simulink model "HDVPSG_DelayComp_NewRef_RealDrop_case1"  (R2019b)
settings: Solver=FixedStepDiscrete  StartTime=0.0  StopTime=28  FixedStep=UT.Ts_Veh  RelTol=1e-3
PostLoadFcn:
  | if any(exist('dsrtsu_mdlpostloadfcn', 'file') ~= 0), dsrtsu_mdlpostloadfcn('Execute', bdroot); end
InitFcn:
  | , if any(exist('dsmpb_private', 'file') ~= 0), dsmpb_private('dsmpb_mdlclblib', 'Init', bdroot); end,
values from neighbouring files (symbols this model uses):
  BETA_HDV_Leader = 50    [HDVPSG_DelayComp_NewRef_RealDrop_script_case1.m]
  BETA_PSG_Follower = 150    [HDVPSG_DelayComp_NewRef_RealDrop_script_case1.m]
  CtrlZone_Length = 250    [HDVPSG_DelayComp_NewRef_RealDrop_script_case1.m]
  DELTA_D_MIN = 5    [HDVPSG_DelayComp_NewRef_RealDrop_script_case1.m]
  DELTA_DR_MG_TCC = 15    [HDVPSG_DelayComp_NewRef_RealDrop_script_case1.m]
  HDV_AMAX = 1.3    [HDVPSG_DelayComp_NewRef_RealDrop_script_case1.m]
  HDV_AMIN = -2.5    [HDVPSG_DelayComp_NewRef_RealDrop_script_case1.m]
  HDV_first_v0 = 13    [HDVPSG_DelayComp_NewRef_RealDrop_script_case1.m]
  HDV_HighMu_D = 9    [HDVPSG_DelayComp_NewRef_RealDrop_script_case1.m]
  HDV_HighMu_I = 27    [HDVPSG_DelayComp_NewRef_RealDrop_script_case1.m]
  HDV_HighMu_P = 27    [HDVPSG_DelayComp_NewRef_RealDrop_script_case1.m]
  HDV_HighMu_TRFC = 0.7    [HDVPSG_DelayComp_NewRef_RealDrop_script_case1.m]
  HDV_last_v0 = 13    [HDVPSG_DelayComp_NewRef_RealDrop_script_case1.m]
  HDV_LowMu_D = 6    [HDVPSG_DelayComp_NewRef_RealDrop_script_case1.m]
  HDV_LowMu_I = 8    [HDVPSG_DelayComp_NewRef_RealDrop_script_case1.m]
  HDV_LowMu_P = 12    [HDVPSG_DelayComp_NewRef_RealDrop_script_case1.m]
  HDV_LowMu_TRFC = 0.6    [HDVPSG_DelayComp_NewRef_RealDrop_script_case1.m]
  Np_MPC = 20    [HDVPSG_DelayComp_NewRef_RealDrop_script_case1.m]
  PSG_AMAX = 3.2    [HDVPSG_DelayComp_NewRef_RealDrop_script_case1.m]
  PSG_AMIN = -6    [HDVPSG_DelayComp_NewRef_RealDrop_script_case1.m]
  PSG_end_v0 = 13    [HDVPSG_DelayComp_NewRef_RealDrop_script_case1.m]
  PSG_first_v0 = 13    [HDVPSG_DelayComp_NewRef_RealDrop_script_case1.m]
  PSG_HighMu_D = 15    [HDVPSG_DelayComp_NewRef_RealDrop_script_case1.m]
  PSG_HighMu_I = 125    [HDVPSG_DelayComp_NewRef_RealDrop_script_case1.m]
  PSG_HighMu_P = 75    [HDVPSG_DelayComp_NewRef_RealDrop_script_case1.m]
  PSG_HighMu_TRFC = 0.8    [HDVPSG_DelayComp_NewRef_RealDrop_script_case1.m]
  PSG_LowMu_D = 12    [HDVPSG_DelayComp_NewRef_RealDrop_script_case1.m]
  PSG_LowMu_I = 64    [HDVPSG_DelayComp_NewRef_RealDrop_script_case1.m]
  PSG_LowMu_P = 48    [HDVPSG_DelayComp_NewRef_RealDrop_script_case1.m]
  PSG_LowMu_TRFC = 0.7    [HDVPSG_DelayComp_NewRef_RealDrop_script_case1.m]
  PSG_middle_v0 = 13    [HDVPSG_DelayComp_NewRef_RealDrop_script_case1.m]
  Q_Leader = 1    [HDVPSG_DelayComp_NewRef_RealDrop_script_case1.m]
  Qd_dot_PSG_Follower = 2    [HDVPSG_DelayComp_NewRef_RealDrop_script_case1.m]
  Qd_PSG_Follower = 10    [HDVPSG_DelayComp_NewRef_RealDrop_script_case1.m]
  R_Leader = 20    [HDVPSG_DelayComp_NewRef_RealDrop_script_case1.m]
  R_PSG_Follower = 1    [HDVPSG_DelayComp_NewRef_RealDrop_script_case1.m]
  Recved_40_1 = Recved_Flag_Combined(47740,:)    [HDVPSG_DelayComp_NewRef_RealDrop_script_case1.m]
  Recved_40_2 = Recved_Flag_Combined(47780,:)    [HDVPSG_DelayComp_NewRef_RealDrop_script_case1.m]
  Recved_40_3 = Recved_Flag_Combined(49536,:)    [HDVPSG_DelayComp_NewRef_RealDrop_script_case1.m]
  Recved_40_4 = Recved_Flag_Combined(118106,:)    [HDVPSG_DelayComp_NewRef_RealDrop_script_case1.m]
  Rho_deltad_PSG_Follower = 1e3    (= 1000)    [HDVPSG_DelayComp_NewRef_RealDrop_script_case1.m]
  Rho_v_PSG_Follower = 1e3    (= 1000)    [HDVPSG_DelayComp_NewRef_RealDrop_script_case1.m]
  T_ADE = 0.01    [HDVPSG_DelayComp_NewRef_RealDrop_script_case1.m]
  V_MAX = 40    [HDVPSG_DelayComp_NewRef_RealDrop_script_case1.m]
  V_MIN = 0    [HDVPSG_DelayComp_NewRef_RealDrop_script_case1.m]
  VR_MG_TCC = 15    [HDVPSG_DelayComp_NewRef_RealDrop_script_case1.m]
undefined symbols (not defined in the file or in its folder): DiscIntNeverNeededParam, UT
libraries: simulink x46
(part 5 of 16)

== system HDVPSG_DelayComp_NewRef_RealDrop_case1/Subsystem1/PSG_first/Global Coordinates ==
  Heading Angle : Inport
  Vx : Inport  Port=2
  Vy : Inport  Port=3
  Add : Sum
  Discrete-Time Integrator : DiscreteIntegrator  SampleTime=UT.Ts_Veh  ICPrevOutput=DiscIntNeverNeededParam  ICPrevScaledInput=DiscIntNeverNeededParam
  Discrete-Time Integrator1 : DiscreteIntegrator  SampleTime=UT.Ts_Veh  ICPrevOutput=DiscIntNeverNeededParam  ICPrevScaledInput=DiscIntNeverNeededParam
  Math Function : Math  Operator=square  SaturateOnIntegerOverflow=on
  Math Function1 : Math  Operator=square  SaturateOnIntegerOverflow=on
  Product{,1..3} (4 alike) : Product
  Sign : Signum
  Sign1 : Signum
  Sqrt : Sqrt  Operator=signedSqrt  SaturateOnIntegerOverflow=on
  Trigonometric Function : Trigonometry
  Trigonometric Function1 : Trigonometry  Operator=cos
  X : Outport  VectorParamsAs1DForOutWhenUnconnected=off
  Y : Outport  Port=2  VectorParamsAs1DForOutWhenUnconnected=off
  wires:
  Product3/1 -> Add/2
  Sign1/1 -> Product3/2
  Math Function1/1 -> Product3/1
  Product2/1 -> Add/1
  Sign/1 -> Product2/2
  Math Function/1 -> Product2/1
  Discrete-Time Integrator/1 -> Y/1
  Discrete-Time Integrator1/1 -> X/1
  Product1/1 -> Discrete-Time Integrator/1
  Product/1 -> Discrete-Time Integrator1/1
  Trigonometric Function/1 -> Product1/1
  Trigonometric Function1/1 -> Product/1
  Sqrt/1 -> Product/2, Product1/2
  Heading Angle/1 -> Trigonometric Function/1, Trigonometric Function1/1
  Add/1 -> Sqrt/1
  Vy/1 -> Sign1/1, Math Function1/1
  Vx/1 -> Sign/1, Math Function/1

== system HDVPSG_DelayComp_NewRef_RealDrop_case1/Subsystem1/PSG_first/left//right wheel steer ==
  steering wheel angle deg : Inport
  Deadband Deg : DeadZone  LowerValue=-2  UpperValue=2  SaturateOnIntegerOverflow=on
  Gain : Gain  Gain=0.9
  Gain1 : Gain  Gain=0.9
  Left wheel rack displacement to ground steering angle1 : Lookup_n-D  NumberOfTableDimensions=1  BreakpointsForDimension1=|  Table=|  RndMeth=Simplest  InputSameDT=on
      | [-83.31
      | -80.10576923
      | -77.13888889
      | -74.38392857
      | -71.81896552
      | -69.425
      | -67.18548387
      | -65.0859375
      | -63.11363636
      | -61.25735294
      | -59.50714286
      | -57.85416667
      | -56.29054054
      | -54.80921053
      | -53.40384615
      | -52.06875
      | -50.79878049
      | -49.58928571
      | -48.43604651
      | -47.33522727
      | -46.28333333
      | -45.27717391
      | -44.31382979
      | -43.390625
      | -42.50510204
      | -41.655
      | 0
      | 41.655
      | 42.50510204
      | 43.390625
      | 44.31382979
      | 45.27717391
      | 46.28333333
      | 47.33522727
      | 48.43604651
      | 49.58928571
      | 50.79878049
      | 52.06875
      | 53.40384615
      | 54.80921053
      | 56.29054054
      | 57.85416667
      | 59.50714286
      | 61.25735294
      | 63.11363636
      | 65.0859375
      | 67.18548387
      | 69.425
      | 71.81896552
      | 74.38392857
      | 77.13888889
      | 80.10576923
      | 83.31
      | ]
      | [-39.37720355
      | -37.63494871
      | -36.07707064
      | -34.67025898
      | -33.38971041
      | -32.21639355
      | -31.13534711
      | -30.13457154
      | -29.20427963
      | -28.33637359
      | -27.52407048
      | -26.76162747
      | -26.04413644
      | -25.36736764
      | -24.72764882
      | -24.12177053
      | -23.54691095
      | -23.00057556
      | -22.48054833
      | -21.98485165
      | -21.51171342
      | -21.05953958
      | -20.62689117
      | -20.21246499
      | -19.81507719
      | -19.43364926
      | 0
      | 23.71741561
      | 24.27669186
      | 24.86323253
      | 25.47909206
      | 26.1265372
      | 26.80807528
      | 27.52648702
      | 28.28486498
      | 29.08665866
      | 29.93572777
      | 30.83640531
      | 31.7935729
      | 32.81275112
      | 33.9002085
      | 35.06309421
      | 36.30960068
      | 37.64916478
      | 39.09271935
      | 40.65301137
      | 42.34501024
      | 44.1864403
      | 46.19848973
      | 48.40677775
      | 50.84271532
      | 53.54549481
      | 56.56514507
      | ]
  Right wheel rack displacement to ground steering angle : Lookup_n-D  NumberOfTableDimensions=1  BreakpointsForDimension1=|  Table=|  RndMeth=Simplest  InputSameDT=on
      | [-83.31
      | -80.10576923
      | -77.13888889
      | -74.38392857
      | -71.81896552
      | -69.425
      | -67.18548387
      | -65.0859375
      | -63.11363636
      | -61.25735294
      | -59.50714286
      | -57.85416667
      | -56.29054054
      | -54.80921053
      | -53.40384615
      | -52.06875
      | -50.79878049
      | -49.58928571
      | -48.43604651
      | -47.33522727
      | -46.28333333
      | -45.27717391
      | -44.31382979
      | -43.390625
      | -42.50510204
      | -41.655
      | 0
      | 41.655
      | 42.50510204
      | 43.390625
      | 44.31382979
      | 45.27717391
      | 46.28333333
      | 47.33522727
      | 48.43604651
      | 49.58928571
      | 50.79878049
      | 52.06875
      | 53.40384615
      | 54.80921053
      | 56.29054054
      | 57.85416667
      | 59.50714286
      | 61.25735294
      | 63.11363636
      | 65.0859375
      | 67.18548387
      | 69.425
      | 71.81896552
      | 74.38392857
      | 77.13888889
      | 80.10576923
      | 83.31
      | ]
      | [-56.56514507
      | -53.54549481
      | -50.84271532
      | -48.40677775
      | -46.19848973
      | -44.1864403
      | -42.34501024
      | -40.65301137
      | -39.09271935
      | -37.64916478
      | -36.30960068
      | -35.06309421
      | -33.9002085
      | -32.81275112
      | -31.7935729
      | -30.83640531
      | -29.93572777
      | -29.08665866
      | -28.28486498
      | -27.52648702
      | -26.80807528
      | -26.1265372
      | -25.47909206
      | -24.86323253
      | -24.27669186
      | -23.71741561
      | 0
      | 19.43364926
      | 19.81507719
      | 20.21246499
      | 20.62689117
      | 21.05953958
      | 21.51171342
      | 21.98485165
      | 22.48054833
      | 23.00057556
      | 23.54691095
      | 24.12177053
      | 24.72764882
      | 25.36736764
      | 26.04413644
      | 26.76162747
      | 27.52407048
      | 28.33637359
      | 29.20427963
      | 30.13457154
      | 31.13534711
      | 32.21639355
      | 33.38971041
      | 34.67025898
      | 36.07707064
      | 37.63494871
      | 39.37720355
      | ]
  steering wheel angle (pinion) to rack dispacement : Lookup_n-D  NumberOfTableDimensions=1  BreakpointsForDimension1=|  Table=|  RndMeth=Simplest  InputSameDT=on
      BreakpointsForDimension1=|
      | [-807.1596203
      | -767.526082
      | -732.1745847
      | -700.3549602
      | -671.5005069
      | -645.1711331
      | -621.017417
      | -598.7568399
      | -578.1574816
      | -559.0264878
      | -541.2017003
      | -524.5454483
      | -508.9398532
      | -494.2832202
      | -480.4872231
      | -467.4746805
      | -455.1777777
      | -443.5366317
      | -432.4981203
      | -422.0149202
      | -412.0447096
      | -402.5495034
      | -393.495094
      | -384.8505798
      | -376.5879637
      | -368.6818104
      | 0
      | 368.6818104
      | 376.5879637
      | 384.8505798
      | 393.495094
      | 402.5495034
      | 412.0447096
      | 422.0149202
      | 432.4981203
      | 443.5366317
      | 455.1777777
      | 467.4746805
      | 480.4872231
      | 494.2832202
      | 508.9398532
      | 524.5454483
      | 541.2017003
      | 559.0264878
      | 578.1574816
      | 598.7568399
      | 621.017417
      | 645.1711331
      | 671.5005069
      | 700.3549602
      | 732.1745847
      | 767.526082
      | 807.1596203
      | ]
      Table=|
      | [-83.31
      | -80.10576923
      | -77.13888889
      | -74.38392857
      | -71.81896552
      | -69.425
      | -67.18548387
      | -65.0859375
      | -63.11363636
      | -61.25735294
      | -59.50714286
      | -57.85416667
      | -56.29054054
      | -54.80921053
      | -53.40384615
      | -52.06875
      | -50.79878049
      | -49.58928571
      | -48.43604651
      | -47.33522727
      | -46.28333333
      | -45.27717391
      | -44.31382979
      | -43.390625
      | -42.50510204
      | -41.655
      | 0
      | 41.655
      | 42.50510204
      | 43.390625
      | 44.31382979
      | 45.27717391
      | 46.28333333
      | 47.33522727
      | 48.43604651
      | 49.58928571
      | 50.79878049
      | 52.06875
      | 53.40384615
      | 54.80921053
      | 56.29054054
      | 57.85416667
      | 59.50714286
      | 61.25735294
      | 63.11363636
      | 65.0859375
      | 67.18548387
      | 69.425
      | 71.81896552
      | 74.38392857
      | 77.13888889
      | 80.10576923
      | 83.31
      | ]
  Right wheel steer ground (deg) : Outport  VectorParamsAs1DForOutWhenUnconnected=off
  Left wheel steer ground (deg) : Outport  Port=2  VectorParamsAs1DForOutWhenUnconnected=off
  wires:
  Deadband Deg/1 -> steering wheel angle (pinion) to rack dispacement/1
  Gain1/1 -> Left wheel steer ground (deg)/1
  Gain/1 -> Right wheel steer ground (deg)/1
  Left wheel rack displacement to ground steering angle1/1 -> Gain1/1
  Right wheel rack displacement to ground steering angle/1 -> Gain/1
  steering wheel angle (pinion) to rack dispacement/1 -> Right wheel rack displacement to ground steering angle/1, Left wheel rack displacement to ground steering angle1/1
  steering wheel angle deg/1 -> Deadband Deg/1

== system HDVPSG_DelayComp_NewRef_RealDrop_case1/Subsystem2/PSG_first/Body Fixed Vehicle Dynamics ==
  Tdf : Inport
  Brake : Inport  Port=2
  deltaFR : Inport  Port=3
  deltaFL : Inport  Port=4
  slope : Inport  Port=5
  TRFC : Inport  Port=6
  V_ini : Inport  Port=7
  yaw_ini : Inport  Port=8
  vy_ini : Inport  Port=9
  8dof_vehicle : Subsystem
  Brakes : Subsystem
  Bus Creator{,2..4} (4 alike) : BusCreator  Inputs=4
  Bus Creator1 : BusCreator  Inputs=8
  Bus Creator5 : BusCreator  Inputs=3
  Bus Selector : BusSelector  OutputSignals=signal1,signal2,signal3,signal4
  Constant : Constant  Value=0
  Constant1 : Constant  Value=0
  Driving Resistance Subsystem : Subsystem
  Fz : Subsystem
  Magic Formula Tire Model1 : Subsystem
  "Tire Longitudinal Center Speed " : Subsystem
  Tire Sideslip Angle : Subsystem
  Unit Delay : UnitDelay  SampleTime=UT.Ts_Veh  HasFrameUpgradeWarning=on
  Unit Delay1 : UnitDelay  SampleTime=UT.Ts_Veh  HasFrameUpgradeWarning=on
  deltaFL1 : InportShadow  Port=4
  deltaFL2 : InportShadow  Port=4
  deltaFR1 : InportShadow  Port=3
  deltaFR2 : InportShadow  Port=3
  lamda slip ratio : Subsystem
  omegafl : Outport  VectorParamsAs1DForOutWhenUnconnected=off
  omegafr : Outport  Port=2  VectorParamsAs1DForOutWhenUnconnected=off
  omegarl : Outport  Port=3  VectorParamsAs1DForOutWhenUnconnected=off
  omegarr : Outport  Port=4  VectorParamsAs1DForOutWhenUnconnected=off
  ax : Outport  Port=5  VectorParamsAs1DForOutWhenUnconnected=off
  Vx : Outport  Port=6  VectorParamsAs1DForOutWhenUnconnected=off
  "Yaw Rate " : Outport  Port=7  VectorParamsAs1DForOutWhenUnconnected=off
  Yaw Angle : Outport  Port=8  VectorParamsAs1DForOutWhenUnconnected=off
  ay : Outport  Port=9  VectorParamsAs1DForOutWhenUnconnected=off
  Vy : Outport  Port=10  VectorParamsAs1DForOutWhenUnconnected=off
  Beta : Outport  Port=11  VectorParamsAs1DForOutWhenUnconnected=off
  Sideslip Angle Alpha : Outport  Port=12  VectorParamsAs1DForOutWhenUnconnected=off
  wires:
  8dof_vehicle/15(Roll Rate) -> Fz/9(roll rate)
  vy_ini/1 -> 8dof_vehicle/14(vy_ini)
  yaw_ini/1 -> 8dof_vehicle/13(yaw_ini)
  V_ini/1 -> 8dof_vehicle/12(V_ini)
  TRFC/1 -> Magic Formula Tire Model1/2(TRFC)
  Bus Creator/1 -> Bus Selector/1
  Tdf/1 -> 8dof_vehicle/1(Tdf)
  8dof_vehicle/1(omegafl) -> omegafl/1, lamda slip ratio/1(omegafl)
  8dof_vehicle/2(omegafr) -> omegafr/1, lamda slip ratio/2(omegafr)
  8dof_vehicle/3(omegarl) -> omegarl/1, lamda slip ratio/3(omegarl)
  8dof_vehicle/4(omegarr) -> omegarr/1, lamda slip ratio/4(omegarr)
  8dof_vehicle/8(Yaw angle) -> Yaw Angle/1
  Bus Creator1/1 -> 8dof_vehicle/6(In7)
  8dof_vehicle/10(Vy) -> Vy/1, Tire Sideslip Angle/1(Vy), "Tire Longitudinal Center Speed "/2(Vy)
  Magic Formula Tire Model1/2(Fy_FL) -> Bus Creator1/2
  Magic Formula Tire Model1/1(Fx_FL) -> Bus Creator1/1
  Fz/4(Fzrr) -> Bus Creator3/4
  Fz/3(Fzrl) -> Bus Creator3/3
  Fz/2(Fzfr) -> Bus Creator3/2
  Fz/1(Fzfl) -> Bus Creator3/1
  Bus Creator2/1 -> Bus Creator5/1, Brakes/1(lambda)  "lamda"
  Bus Creator4/1 -> Bus Creator5/3  "alpha"
  Bus Creator5/1 -> Magic Formula Tire Model1/1(VehState)
  Tire Sideslip Angle/4(alpha_rr: rad) -> Bus Creator4/4
  Tire Sideslip Angle/3(alpha_rl: rad) -> Bus Creator4/3
  Tire Sideslip Angle/1(alpha_fl: rad) -> Bus Creator4/1, Sideslip Angle Alpha/1
  Tire Sideslip Angle/2(alpha_fr: rad) -> Bus Creator4/2
  "Tire Longitudinal Center Speed "/4(Vwrr) -> Bus Creator/4
  "Tire Longitudinal Center Speed "/2(Vwfr) -> Bus Creator/2
  "Tire Longitudinal Center Speed "/1(Vwfl) -> Bus Creator/1
  "Tire Longitudinal Center Speed "/3(Vwrl) -> Bus Creator/3
  Bus Selector/1 -> lamda slip ratio/5(Vwfl)  "<signal1>"
  Bus Selector/2 -> lamda slip ratio/6(Vwfr)  "<signal2>"
  Bus Selector/3 -> lamda slip ratio/7(Vwrl)  "<signal3>"
  Bus Selector/4 -> lamda slip ratio/8(Vwrr)  "<signal4>"
  Driving Resistance Subsystem/2(Fr) -> 8dof_vehicle/8(Fr)
  deltaFL/1 -> lamda slip ratio/9(deltaFL)  "deltaw"
  deltaFL1/1 -> Tire Sideslip Angle/4(deltaFL)  "deltaw"
  8dof_vehicle/9(ay) -> ay/1, Unit Delay1/1
  8dof_vehicle/11("Veh Sideslip, Beta") -> "Tire Longitudinal Center Speed "/4(VehSideSlip Beta), Beta/1, Tire Sideslip Angle/6(Beta)
  8dof_vehicle/6(Vx) -> Vx/1, Driving Resistance Subsystem/1(Vx), Tire Sideslip Angle/3(Vx), "Tire Longitudinal Center Speed "/1(Vx)
  8dof_vehicle/7(Yaw Rate) -> "Yaw Rate "/1, Tire Sideslip Angle/2(Yaw Rate), "Tire Longitudinal Center Speed "/3(YawRate)
  slope/1 -> 8dof_vehicle/9(slope)
  Constant1/1 -> Fz/6(bank angle)
  Driving Resistance Subsystem/1(Fax) -> Fz/1(Fa), 8dof_vehicle/7(Fax)
  Constant/1 -> Fz/3(slope)
  8dof_vehicle/5(ax) -> ax/1, Unit Delay/1
  deltaFL2/1 -> 8dof_vehicle/10(deltaFL)  "deltaw"
  Magic Formula Tire Model1/5(Fx_RL) -> Bus Creator1/5
  Magic Formula Tire Model1/7(Fx_RR) -> Bus Creator1/7
  Magic Formula Tire Model1/8(Fy_RR) -> Bus Creator1/8
  Magic Formula Tire Model1/6(Fy_RL) -> Bus Creator1/6
  Magic Formula Tire Model1/3(Fx_FR) -> Bus Creator1/3
  Magic Formula Tire Model1/4(Fy_FR) -> Bus Creator1/4
  Unit Delay1/1 -> Fz/5(ay)
  Unit Delay/1 -> Fz/2(ax)
  lamda slip ratio/1(lamdafl) -> Bus Creator2/1
  lamda slip ratio/2(lamdafr) -> Bus Creator2/2
  lamda slip ratio/3(lamdarl) -> Bus Creator2/3
  lamda slip ratio/4(lamdarr) -> Bus Creator2/4
  deltaFR/1 -> lamda slip ratio/10(deltaFR)
  deltaFR1/1 -> Tire Sideslip Angle/5(deltaFR1)
  deltaFR2/1 -> 8dof_vehicle/11(deltaRL)
  Bus Creator3/1 -> Bus Creator5/2
  8dof_vehicle/13(Pitch_rate) -> Fz/8(pitch rate)
  8dof_vehicle/12(Pitch) -> Fz/4(pitch angle)
  8dof_vehicle/14("Roll ") -> Fz/7(roll angle)
  Brake/1 -> Brakes/2(brake postion)
  Brakes/1(Tbfl) -> 8dof_vehicle/2(Tbfl)
  Brakes/2(Tbfr) -> 8dof_vehicle/3(Tbfr)
  Brakes/3(Tbrl) -> 8dof_vehicle/4(Tbrl)
  Brakes/4(Tbrr) -> 8dof_vehicle/5(Tbrr)

== system HDVPSG_DelayComp_NewRef_RealDrop_case1/Subsystem2/PSG_first/Cruise Speed Control ==
  Vx : Inport
  Vxr : Inport  Port=2
  PID_P : Inport  Port=3
  PID_I : Inport  Port=4
  PID_D : Inport  Port=5
  Constant : Constant  Value=100
  Gain : Gain  Gain=2
  PID Controller : simulink/Continuous/PID Controller  Controller=PID  Form=Parallel  TimeDomain=Discrete-time  SampleTime=UT.Ts_Veh  IntegratorMethod=Forward Euler  FilterMethod=Forward Euler  ControllerParametersSource=external  P=UT.PID_P_PSG  I=UT.PID_I_PSG  D=UT.PID_D_PSG  UseFilter=on  N=100  TunerSelectOption=Transfer Function Based (PID Tuner App)  InitialConditionSource=internal  InitialConditionForIntegrator=0  InitialConditionForFilter=0  DifferentiatorICPrevScaledInput=0  ExternalReset=none  TrackingMode=off  Kt=1  LimitOutput=off  UpperSaturationLimit=inf  LowerSaturationLimit=-inf  LinearizeAsGain=on  AntiWindupMode=none  Kb=1  POutMin=[]  POutMax=[]  IOutMin=[]  IOutMax=[]  DOutMin=[]  DOutMax=[]  NOutMin=[]  NOutMax=[]  SumOutMin=[]  SumOutMax=[]  SaturationOutMin=[]  SaturationOutMax=[]  PParamMin=[]  PParamMax=[]  IParamMin=[]  IParamMax=[]  DParamMin=[]  DParamMax=[]  NParamMin=[]  NParamMax=[]  KbParamMin=[]  KbParamMax=[]  KtParamMin=[]  KtParamMax=[]  KbOutMin=[]  KbOutMax=[]  KtOutMin=[]  KtOutMax=[]  IntegratorOutMin=[]  IntegratorOutMax=[]  FilterOutMin=[]  FilterOutMax=[]  SumI1OutMin=[]  SumI1OutMax=[]  SumI2OutMin=[]  SumI2OutMax=[]  SumI3OutMin=[]  SumI3OutMax=[]  SumI4OutMin=[]  SumI4OutMax=[]  SumDOutMin=[]  SumDOutMax=[]  DifferentiatorOutMin=[]  DifferentiatorOutMax=[]  FilterDiffOutCoefMin=[]  FilterDiffOutCoefMax=[]  ReciprocalOutMin=[]  ReciprocalOutMax=[]  SumDenOutMin=[]  SumDenOutMax=[]  SumNumOutMin=[]  SumNumOutMax=[]  DivideOutMin=[]  DivideOutMax=[]  IntegratorContinuousStateAttributes=''  IntegratorStateMustResolveToSignalObject=off  IntegratorRTWStateStorageClass=Auto  FilterContinuousStateAttributes=''  FilterStateMustResolveToSignalObject=off  FilterRTWStateStorageClass=Auto  ParallelPVariant=ExternalParameters  IdealPVariant=Disabled  IVariant=ExternalParameters  DVariant=ExternalParameters  IntegratorVariant=Discrete  SatVariant=Disabled  AWVariant=Passthrough  PCopyVariant=Disabled  TRVariant=Disabled  FdbkBlocksVariant=Forward  IdealPFdbkVariant=Disabled  SatFdbkVariant=Disabled  DerivativeFilterVariant=ForwardEulerFilter  NVariant=ExternalParameters  NCopyVariant=Disabled  FilterICVariant=InternalICsFilter  IntegratorICVariant=InternalICs  ExternalResetVariant=Disabled  TRSumVariant=Passthrough  SumFdbkVariant=Disabled  SumVariant=Sum_PID
  Subtract : Sum  Inputs=-+
  Throttle : Outport  VectorParamsAs1DForOutWhenUnconnected=off
  wires:
  PID_D/1 -> PID Controller/4
  PID_I/1 -> PID Controller/3
  PID_P/1 -> PID Controller/2
  Constant/1 -> PID Controller/5
  PID Controller/1 -> Gain/1
  Subtract/1 -> PID Controller/1
  Gain/1 -> Throttle/1
  Vxr/1 -> Subtract/2
  Vx/1 -> Subtract/1

== system HDVPSG_DelayComp_NewRef_RealDrop_case1/Subsystem2/PSG_first/Global Coordinates ==
  Heading Angle : Inport
  Vx : Inport  Port=2
  Vy : Inport  Port=3
  Add : Sum
  Discrete-Time Integrator : DiscreteIntegrator  SampleTime=UT.Ts_Veh  ICPrevOutput=DiscIntNeverNeededParam  ICPrevScaledInput=DiscIntNeverNeededParam
  Discrete-Time Integrator1 : DiscreteIntegrator  SampleTime=UT.Ts_Veh  ICPrevOutput=DiscIntNeverNeededParam  ICPrevScaledInput=DiscIntNeverNeededParam
  Math Function : Math  Operator=square  SaturateOnIntegerOverflow=on
  Math Function1 : Math  Operator=square  SaturateOnIntegerOverflow=on
  Product{,1..3} (4 alike) : Product
  Sign : Signum
  Sign1 : Signum
  Sqrt : Sqrt  Operator=signedSqrt  SaturateOnIntegerOverflow=on
  Trigonometric Function : Trigonometry
  Trigonometric Function1 : Trigonometry  Operator=cos
  X : Outport  VectorParamsAs1DForOutWhenUnconnected=off
  Y : Outport  Port=2  VectorParamsAs1DForOutWhenUnconnected=off
  wires:
  Vx/1 -> Math Function/1, Sign/1
  Vy/1 -> Math Function1/1, Sign1/1
  Add/1 -> Sqrt/1
  Heading Angle/1 -> Trigonometric Function1/1, Trigonometric Function/1
  Sqrt/1 -> Product1/2, Product/2
  Trigonometric Function1/1 -> Product/1
  Trigonometric Function/1 -> Product1/1
  Product/1 -> Discrete-Time Integrator1/1
  Product1/1 -> Discrete-Time Integrator/1
  Discrete-Time Integrator1/1 -> X/1
  Discrete-Time Integrator/1 -> Y/1
  Math Function/1 -> Product2/1
  Sign/1 -> Product2/2
  Product2/1 -> Add/1
  Math Function1/1 -> Product3/1
  Sign1/1 -> Product3/2
  Product3/1 -> Add/2

== system HDVPSG_DelayComp_NewRef_RealDrop_case1/Subsystem2/PSG_first/left//right wheel steer ==
  steering wheel angle deg : Inport
  Deadband Deg : DeadZone  LowerValue=-2  UpperValue=2  SaturateOnIntegerOverflow=on
  Gain : Gain  Gain=0.9
  Gain1 : Gain  Gain=0.9
  Left wheel rack displacement to ground steering angle1 : Lookup_n-D  NumberOfTableDimensions=1  BreakpointsForDimension1=|  Table=|  RndMeth=Simplest  InputSameDT=on
      | [-83.31
      | -80.10576923
      | -77.13888889
      | -74.38392857
      | -71.81896552
      | -69.425
      | -67.18548387
      | -65.0859375
      | -63.11363636
      | -61.25735294
      | -59.50714286
      | -57.85416667
      | -56.29054054
      | -54.80921053
      | -53.40384615
      | -52.06875
      | -50.79878049
      | -49.58928571
      | -48.43604651
      | -47.33522727
      | -46.28333333
      | -45.27717391
      | -44.31382979
      | -43.390625
      | -42.50510204
      | -41.655
      | 0
      | 41.655
      | 42.50510204
      | 43.390625
      | 44.31382979
      | 45.27717391
      | 46.28333333
      | 47.33522727
      | 48.43604651
      | 49.58928571
      | 50.79878049
      | 52.06875
      | 53.40384615
      | 54.80921053
      | 56.29054054
      | 57.85416667
      | 59.50714286
      | 61.25735294
      | 63.11363636
      | 65.0859375
      | 67.18548387
      | 69.425
      | 71.81896552
      | 74.38392857
      | 77.13888889
      | 80.10576923
      | 83.31
      | ]
      | [-39.37720355
      | -37.63494871
      | -36.07707064
      | -34.67025898
      | -33.38971041
      | -32.21639355
      | -31.13534711
      | -30.13457154
      | -29.20427963
      | -28.33637359
      | -27.52407048
      | -26.76162747
      | -26.04413644
      | -25.36736764
      | -24.72764882
      | -24.12177053
      | -23.54691095
      | -23.00057556
      | -22.48054833
      | -21.98485165
      | -21.51171342
      | -21.05953958
      | -20.62689117
      | -20.21246499
      | -19.81507719
      | -19.43364926
      | 0
      | 23.71741561
      | 24.27669186
      | 24.86323253
      | 25.47909206
      | 26.1265372
      | 26.80807528
      | 27.52648702
      | 28.28486498
      | 29.08665866
      | 29.93572777
      | 30.83640531
      | 31.7935729
      | 32.81275112
      | 33.9002085
      | 35.06309421
      | 36.30960068
      | 37.64916478
      | 39.09271935
      | 40.65301137
      | 42.34501024
      | 44.1864403
      | 46.19848973
      | 48.40677775
      | 50.84271532
      | 53.54549481
      | 56.56514507
      | ]
  Right wheel rack displacement to ground steering angle : Lookup_n-D  NumberOfTableDimensions=1  BreakpointsForDimension1=|  Table=|  RndMeth=Simplest  InputSameDT=on
      | [-83.31
      | -80.10576923
      | -77.13888889
      | -74.38392857
      | -71.81896552
      | -69.425
      | -67.18548387
      | -65.0859375
      | -63.11363636
      | -61.25735294
      | -59.50714286
      | -57.85416667
      | -56.29054054
      | -54.80921053
      | -53.40384615
      | -52.06875
      | -50.79878049
      | -49.58928571
      | -48.43604651
      | -47.33522727
      | -46.28333333
      | -45.27717391
      | -44.31382979
      | -43.390625
      | -42.50510204
      | -41.655
      | 0
      | 41.655
      | 42.50510204
      | 43.390625
      | 44.31382979
      | 45.27717391
      | 46.28333333
      | 47.33522727
      | 48.43604651
      | 49.58928571
      | 50.79878049
      | 52.06875
      | 53.40384615
      | 54.80921053
      | 56.29054054
      | 57.85416667
      | 59.50714286
      | 61.25735294
      | 63.11363636
      | 65.0859375
      | 67.18548387
      | 69.425
      | 71.81896552
      | 74.38392857
      | 77.13888889
      | 80.10576923
      | 83.31
      | ]
      | [-56.56514507
      | -53.54549481
      | -50.84271532
      | -48.40677775
      | -46.19848973
      | -44.1864403
      | -42.34501024
      | -40.65301137
      | -39.09271935
      | -37.64916478
      | -36.30960068
      | -35.06309421
      | -33.9002085
      | -32.81275112
      | -31.7935729
      | -30.83640531
      | -29.93572777
      | -29.08665866
      | -28.28486498
      | -27.52648702
      | -26.80807528
      | -26.1265372
      | -25.47909206
      | -24.86323253
      | -24.27669186
      | -23.71741561
      | 0
      | 19.43364926
      | 19.81507719
      | 20.21246499
      | 20.62689117
      | 21.05953958
      | 21.51171342
      | 21.98485165
      | 22.48054833
      | 23.00057556
      | 23.54691095
      | 24.12177053
      | 24.72764882
      | 25.36736764
      | 26.04413644
      | 26.76162747
      | 27.52407048
      | 28.33637359
      | 29.20427963
      | 30.13457154
      | 31.13534711
      | 32.21639355
      | 33.38971041
      | 34.67025898
      | 36.07707064
      | 37.63494871
      | 39.37720355
      | ]
  steering wheel angle (pinion) to rack dispacement : Lookup_n-D  NumberOfTableDimensions=1  BreakpointsForDimension1=|  Table=|  RndMeth=Simplest  InputSameDT=on
      BreakpointsForDimension1=|
      | [-807.1596203
      | -767.526082
      | -732.1745847
      | -700.3549602
      | -671.5005069
      | -645.1711331
      | -621.017417
      | -598.7568399
      | -578.1574816
      | -559.0264878
      | -541.2017003
      | -524.5454483
      | -508.9398532
      | -494.2832202
      | -480.4872231
      | -467.4746805
      | -455.1777777
      | -443.5366317
      | -432.4981203
      | -422.0149202
      | -412.0447096
      | -402.5495034
      | -393.495094
      | -384.8505798
      | -376.5879637
      | -368.6818104
      | 0
      | 368.6818104
      | 376.5879637
      | 384.8505798
      | 393.495094
      | 402.5495034
      | 412.0447096
      | 422.0149202
      | 432.4981203
      | 443.5366317
      | 455.1777777
      | 467.4746805
      | 480.4872231
      | 494.2832202
      | 508.9398532
      | 524.5454483
      | 541.2017003
      | 559.0264878
      | 578.1574816
      | 598.7568399
      | 621.017417
      | 645.1711331
      | 671.5005069
      | 700.3549602
      | 732.1745847
      | 767.526082
      | 807.1596203
      | ]
      Table=|
      | [-83.31
      | -80.10576923
      | -77.13888889
      | -74.38392857
      | -71.81896552
      | -69.425
      | -67.18548387
      | -65.0859375
      | -63.11363636
      | -61.25735294
      | -59.50714286
      | -57.85416667
      | -56.29054054
      | -54.80921053
      | -53.40384615
      | -52.06875
      | -50.79878049
      | -49.58928571
      | -48.43604651
      | -47.33522727
      | -46.28333333
      | -45.27717391
      | -44.31382979
      | -43.390625
      | -42.50510204
      | -41.655
      | 0
      | 41.655
      | 42.50510204
      | 43.390625
      | 44.31382979
      | 45.27717391
      | 46.28333333
      | 47.33522727
      | 48.43604651
      | 49.58928571
      | 50.79878049
      | 52.06875
      | 53.40384615
      | 54.80921053
      | 56.29054054
      | 57.85416667
      | 59.50714286
      | 61.25735294
      | 63.11363636
      | 65.0859375
      | 67.18548387
      | 69.425
      | 71.81896552
      | 74.38392857
      | 77.13888889
      | 80.10576923
      | 83.31
      | ]
  Right wheel steer ground (deg) : Outport  VectorParamsAs1DForOutWhenUnconnected=off
  Left wheel steer ground (deg) : Outport  Port=2  VectorParamsAs1DForOutWhenUnconnected=off
  wires:
  steering wheel angle deg/1 -> Deadband Deg/1
  steering wheel angle (pinion) to rack dispacement/1 -> Left wheel rack displacement to ground steering angle1/1, Right wheel rack displacement to ground steering angle/1
  Right wheel rack displacement to ground steering angle/1 -> Gain/1
  Left wheel rack displacement to ground steering angle1/1 -> Gain1/1
  Gain/1 -> Right wheel steer ground (deg)/1
  Gain1/1 -> Left wheel steer ground (deg)/1
  Deadband Deg/1 -> steering wheel angle (pinion) to rack dispacement/1

== system HDVPSG_DelayComp_NewRef_RealDrop_case1/Subsystem29/PSG_first/Body Fixed Vehicle Dynamics ==
  Tdf : Inport
  Brake : Inport  Port=2
  deltaFR : Inport  Port=3
  deltaFL : Inport  Port=4
  slope : Inport  Port=5
  TRFC : Inport  Port=6
  V_ini : Inport  Port=7
  yaw_ini : Inport  Port=8
  vy_ini : Inport  Port=9
  8dof_vehicle : Subsystem
  Brakes : Subsystem
  Bus Creator{,2..4} (4 alike) : BusCreator  Inputs=4
  Bus Creator1 : BusCreator  Inputs=8
  Bus Creator5 : BusCreator  Inputs=3
  Bus Selector : BusSelector  OutputSignals=signal1,signal2,signal3,signal4
  Constant : Constant  Value=0
  Constant1 : Constant  Value=0
  Driving Resistance Subsystem : Subsystem
  Fz : Subsystem
  Magic Formula Tire Model1 : Subsystem
  "Tire Longitudinal Center Speed " : Subsystem
  Tire Sideslip Angle : Subsystem
  To Workspace : ToWorkspace  VariableName=PSG1_FxFL  SaveFormat=Timeseries  SampleTime=-1
  To Workspace1 : ToWorkspace  VariableName=PSG1_FxRL  SaveFormat=Timeseries  SampleTime=-1
  To Workspace2 : ToWorkspace  VariableName=PSG1_FxFR  SaveFormat=Timeseries  SampleTime=-1
  To Workspace3 : ToWorkspace  VariableName=PSG1_FxRR  SaveFormat=Timeseries  SampleTime=-1
  Unit Delay : UnitDelay  SampleTime=UT.Ts_Veh  HasFrameUpgradeWarning=on
  Unit Delay1 : UnitDelay  SampleTime=UT.Ts_Veh  HasFrameUpgradeWarning=on
  deltaFL1 : InportShadow  Port=4
  deltaFL2 : InportShadow  Port=4
  deltaFR1 : InportShadow  Port=3
  deltaFR2 : InportShadow  Port=3
  lamda slip ratio : Subsystem
  omegafl : Outport  VectorParamsAs1DForOutWhenUnconnected=off
  omegafr : Outport  Port=2  VectorParamsAs1DForOutWhenUnconnected=off
  omegarl : Outport  Port=3  VectorParamsAs1DForOutWhenUnconnected=off
  omegarr : Outport  Port=4  VectorParamsAs1DForOutWhenUnconnected=off
  ax : Outport  Port=5  VectorParamsAs1DForOutWhenUnconnected=off
  Vx : Outport  Port=6  VectorParamsAs1DForOutWhenUnconnected=off
  "Yaw Rate " : Outport  Port=7  VectorParamsAs1DForOutWhenUnconnected=off
  Yaw Angle : Outport  Port=8  VectorParamsAs1DForOutWhenUnconnected=off
  ay : Outport  Port=9  VectorParamsAs1DForOutWhenUnconnected=off
  Vy : Outport  Port=10  VectorParamsAs1DForOutWhenUnconnected=off
  Beta : Outport  Port=11  VectorParamsAs1DForOutWhenUnconnected=off
  Sideslip Angle Alpha : Outport  Port=12  VectorParamsAs1DForOutWhenUnconnected=off
  wires:
  8dof_vehicle/15(Roll Rate) -> Fz/9(roll rate)
  vy_ini/1 -> 8dof_vehicle/14(vy_ini)
  yaw_ini/1 -> 8dof_vehicle/13(yaw_ini)
  V_ini/1 -> 8dof_vehicle/12(V_ini)
  TRFC/1 -> Magic Formula Tire Model1/2(TRFC)
  Bus Creator/1 -> Bus Selector/1
  Tdf/1 -> 8dof_vehicle/1(Tdf)
  8dof_vehicle/1(omegafl) -> omegafl/1, lamda slip ratio/1(omegafl)
  8dof_vehicle/2(omegafr) -> omegafr/1, lamda slip ratio/2(omegafr)
  8dof_vehicle/3(omegarl) -> omegarl/1, lamda slip ratio/3(omegarl)
  8dof_vehicle/4(omegarr) -> omegarr/1, lamda slip ratio/4(omegarr)
  8dof_vehicle/8(Yaw angle) -> Yaw Angle/1
  Bus Creator1/1 -> 8dof_vehicle/6(In7)
  8dof_vehicle/10(Vy) -> Vy/1, Tire Sideslip Angle/1(Vy), "Tire Longitudinal Center Speed "/2(Vy)
  Magic Formula Tire Model1/2(Fy_FL) -> Bus Creator1/2
  Magic Formula Tire Model1/1(Fx_FL) -> To Workspace/1, Bus Creator1/1
  Fz/4(Fzrr) -> Bus Creator3/4
  Fz/3(Fzrl) -> Bus Creator3/3
  Fz/2(Fzfr) -> Bus Creator3/2
  Fz/1(Fzfl) -> Bus Creator3/1
  Bus Creator2/1 -> Bus Creator5/1, Brakes/1(lambda)  "lamda"
  Bus Creator4/1 -> Bus Creator5/3  "alpha"
  Bus Creator5/1 -> Magic Formula Tire Model1/1(VehState)
  Tire Sideslip Angle/4(alpha_rr: rad) -> Bus Creator4/4
  Tire Sideslip Angle/3(alpha_rl: rad) -> Bus Creator4/3
  Tire Sideslip Angle/1(alpha_fl: rad) -> Bus Creator4/1, Sideslip Angle Alpha/1
  Tire Sideslip Angle/2(alpha_fr: rad) -> Bus Creator4/2
  "Tire Longitudinal Center Speed "/4(Vwrr) -> Bus Creator/4
  "Tire Longitudinal Center Speed "/2(Vwfr) -> Bus Creator/2
  "Tire Longitudinal Center Speed "/1(Vwfl) -> Bus Creator/1
  "Tire Longitudinal Center Speed "/3(Vwrl) -> Bus Creator/3
  Bus Selector/1 -> lamda slip ratio/5(Vwfl)  "<signal1>"
  Bus Selector/2 -> lamda slip ratio/6(Vwfr)  "<signal2>"
  Bus Selector/3 -> lamda slip ratio/7(Vwrl)  "<signal3>"
  Bus Selector/4 -> lamda slip ratio/8(Vwrr)  "<signal4>"
  Driving Resistance Subsystem/2(Fr) -> 8dof_vehicle/8(Fr)
  deltaFL/1 -> lamda slip ratio/9(deltaFL)  "deltaw"
  deltaFL1/1 -> Tire Sideslip Angle/4(deltaFL)  "deltaw"
  8dof_vehicle/9(ay) -> ay/1, Unit Delay1/1
  8dof_vehicle/11("Veh Sideslip, Beta") -> "Tire Longitudinal Center Speed "/4(VehSideSlip Beta), Beta/1, Tire Sideslip Angle/6(Beta)
  8dof_vehicle/6(Vx) -> Vx/1, Driving Resistance Subsystem/1(Vx), Tire Sideslip Angle/3(Vx), "Tire Longitudinal Center Speed "/1(Vx)
  8dof_vehicle/7(Yaw Rate) -> "Yaw Rate "/1, Tire Sideslip Angle/2(Yaw Rate), "Tire Longitudinal Center Speed "/3(YawRate)
  slope/1 -> 8dof_vehicle/9(slope)
  Constant1/1 -> Fz/6(bank angle)
  Driving Resistance Subsystem/1(Fax) -> Fz/1(Fa), 8dof_vehicle/7(Fax)
  Constant/1 -> Fz/3(slope)
  8dof_vehicle/5(ax) -> ax/1, Unit Delay/1
  deltaFL2/1 -> 8dof_vehicle/10(deltaFL)  "deltaw"
  Magic Formula Tire Model1/5(Fx_RL) -> To Workspace1/1, Bus Creator1/5
  Magic Formula Tire Model1/7(Fx_RR) -> To Workspace3/1, Bus Creator1/7
  Magic Formula Tire Model1/8(Fy_RR) -> Bus Creator1/8
  Magic Formula Tire Model1/6(Fy_RL) -> Bus Creator1/6
  Magic Formula Tire Model1/3(Fx_FR) -> To Workspace2/1, Bus Creator1/3
  Magic Formula Tire Model1/4(Fy_FR) -> Bus Creator1/4
  Unit Delay1/1 -> Fz/5(ay)
  Unit Delay/1 -> Fz/2(ax)
  lamda slip ratio/1(lamdafl) -> Bus Creator2/1
  lamda slip ratio/2(lamdafr) -> Bus Creator2/2
  lamda slip ratio/3(lamdarl) -> Bus Creator2/3
  lamda slip ratio/4(lamdarr) -> Bus Creator2/4
  deltaFR/1 -> lamda slip ratio/10(deltaFR)
  deltaFR1/1 -> Tire Sideslip Angle/5(deltaFR1)
  deltaFR2/1 -> 8dof_vehicle/11(deltaRL)
  Bus Creator3/1 -> Bus Creator5/2
  8dof_vehicle/13(Pitch_rate) -> Fz/8(pitch rate)
  8dof_vehicle/12(Pitch) -> Fz/4(pitch angle)
  8dof_vehicle/14("Roll ") -> Fz/7(roll angle)
  Brake/1 -> Brakes/2(brake postion)
  Brakes/1(Tbfl) -> 8dof_vehicle/2(Tbfl)
  Brakes/2(Tbfr) -> 8dof_vehicle/3(Tbfr)
  Brakes/3(Tbrl) -> 8dof_vehicle/4(Tbrl)
  Brakes/4(Tbrr) -> 8dof_vehicle/5(Tbrr)

== system HDVPSG_DelayComp_NewRef_RealDrop_case1/Subsystem29/PSG_first/Cruise Speed Control ==
  Vx : Inport
  Vxr : Inport  Port=2
  PID_P : Inport  Port=3
  PID_I : Inport  Port=4
  PID_D : Inport  Port=5
  Constant : Constant  Value=100
  Gain : Gain  Gain=2
  PID Controller : simulink/Continuous/PID Controller  Controller=PID  Form=Parallel  TimeDomain=Discrete-time  SampleTime=UT.Ts_Veh  IntegratorMethod=Forward Euler  FilterMethod=Forward Euler  ControllerParametersSource=external  P=UT.PID_P_PSG  I=UT.PID_I_PSG  D=UT.PID_D_PSG  UseFilter=on  N=100  TunerSelectOption=Transfer Function Based (PID Tuner App)  InitialConditionSource=internal  InitialConditionForIntegrator=0  InitialConditionForFilter=0  DifferentiatorICPrevScaledInput=0  ExternalReset=none  TrackingMode=off  Kt=1  LimitOutput=off  UpperSaturationLimit=inf  LowerSaturationLimit=-inf  LinearizeAsGain=on  AntiWindupMode=none  Kb=1  POutMin=[]  POutMax=[]  IOutMin=[]  IOutMax=[]  DOutMin=[]  DOutMax=[]  NOutMin=[]  NOutMax=[]  SumOutMin=[]  SumOutMax=[]  SaturationOutMin=[]  SaturationOutMax=[]  PParamMin=[]  PParamMax=[]  IParamMin=[]  IParamMax=[]  DParamMin=[]  DParamMax=[]  NParamMin=[]  NParamMax=[]  KbParamMin=[]  KbParamMax=[]  KtParamMin=[]  KtParamMax=[]  KbOutMin=[]  KbOutMax=[]  KtOutMin=[]  KtOutMax=[]  IntegratorOutMin=[]  IntegratorOutMax=[]  FilterOutMin=[]  FilterOutMax=[]  SumI1OutMin=[]  SumI1OutMax=[]  SumI2OutMin=[]  SumI2OutMax=[]  SumI3OutMin=[]  SumI3OutMax=[]  SumI4OutMin=[]  SumI4OutMax=[]  SumDOutMin=[]  SumDOutMax=[]  DifferentiatorOutMin=[]  DifferentiatorOutMax=[]  FilterDiffOutCoefMin=[]  FilterDiffOutCoefMax=[]  ReciprocalOutMin=[]  ReciprocalOutMax=[]  SumDenOutMin=[]  SumDenOutMax=[]  SumNumOutMin=[]  SumNumOutMax=[]  DivideOutMin=[]  DivideOutMax=[]  IntegratorContinuousStateAttributes=''  IntegratorStateMustResolveToSignalObject=off  IntegratorRTWStateStorageClass=Auto  FilterContinuousStateAttributes=''  FilterStateMustResolveToSignalObject=off  FilterRTWStateStorageClass=Auto  ParallelPVariant=ExternalParameters  IdealPVariant=Disabled  IVariant=ExternalParameters  DVariant=ExternalParameters  IntegratorVariant=Discrete  SatVariant=Disabled  AWVariant=Passthrough  PCopyVariant=Disabled  TRVariant=Disabled  FdbkBlocksVariant=Forward  IdealPFdbkVariant=Disabled  SatFdbkVariant=Disabled  DerivativeFilterVariant=ForwardEulerFilter  NVariant=ExternalParameters  NCopyVariant=Disabled  FilterICVariant=InternalICsFilter  IntegratorICVariant=InternalICs  ExternalResetVariant=Disabled  TRSumVariant=Passthrough  SumFdbkVariant=Disabled  SumVariant=Sum_PID
  Subtract : Sum  Inputs=-+
  Throttle : Outport  VectorParamsAs1DForOutWhenUnconnected=off
  wires:
  PID_D/1 -> PID Controller/4
  PID_I/1 -> PID Controller/3
  PID_P/1 -> PID Controller/2
  Constant/1 -> PID Controller/5
  PID Controller/1 -> Gain/1
  Subtract/1 -> PID Controller/1
  Gain/1 -> Throttle/1
  Vxr/1 -> Subtract/2
  Vx/1 -> Subtract/1

== system HDVPSG_DelayComp_NewRef_RealDrop_case1/Subsystem29/PSG_first/Global Coordinates ==
  Heading Angle : Inport
  Vx : Inport  Port=2
  Vy : Inport  Port=3
  Add : Sum
  Discrete-Time Integrator : DiscreteIntegrator  SampleTime=UT.Ts_Veh  ICPrevOutput=DiscIntNeverNeededParam  ICPrevScaledInput=DiscIntNeverNeededParam
  Discrete-Time Integrator1 : DiscreteIntegrator  SampleTime=UT.Ts_Veh  ICPrevOutput=DiscIntNeverNeededParam  ICPrevScaledInput=DiscIntNeverNeededParam
  Math Function : Math  Operator=square  SaturateOnIntegerOverflow=on
  Math Function1 : Math  Operator=square  SaturateOnIntegerOverflow=on
  Product{,1..3} (4 alike) : Product
  Sign : Signum
  Sign1 : Signum
  Sqrt : Sqrt  Operator=signedSqrt  SaturateOnIntegerOverflow=on
  Trigonometric Function : Trigonometry
  Trigonometric Function1 : Trigonometry  Operator=cos
  X : Outport  VectorParamsAs1DForOutWhenUnconnected=off
  Y : Outport  Port=2  VectorParamsAs1DForOutWhenUnconnected=off
  wires:
  Vx/1 -> Math Function/1, Sign/1
  Vy/1 -> Math Function1/1, Sign1/1
  Add/1 -> Sqrt/1
  Heading Angle/1 -> Trigonometric Function1/1, Trigonometric Function/1
  Sqrt/1 -> Product1/2, Product/2
  Trigonometric Function1/1 -> Product/1
  Trigonometric Function/1 -> Product1/1
  Product/1 -> Discrete-Time Integrator1/1
  Product1/1 -> Discrete-Time Integrator/1
  Discrete-Time Integrator1/1 -> X/1
  Discrete-Time Integrator/1 -> Y/1
  Math Function/1 -> Product2/1
  Sign/1 -> Product2/2
  Product2/1 -> Add/1
  Math Function1/1 -> Product3/1
  Sign1/1 -> Product3/2
  Product3/1 -> Add/2
